simulink model "PubIfDecisionTOS_MDL"  (R2020b)
settings: configuration reference "DspaceConfig" (kept outside this file)
PostLoadFcn:
  | if any(exist('dsrtsu_mdlpostloadfcn', 'file') ~= 0), dsrtsu_mdlpostloadfcn('Execute', bdroot); end
InitFcn:
  | , if any(exist('dsmpb_private', 'file') ~= 0), dsmpb_private('dsmpb_mdlclblib', 'Init', bdroot); end,
undefined symbols (not defined in the file or in its folder): C_TOS_ACCEgoRAxletoFbumplength_m, C_TOS_ACCTargetFront_Flag, C_TOS_AEBJAPedObjDxThre_Val, C_TOS_AEBJAPedObjDyThre_Val, C_TOS_AEBJATargetSize_Val, C_TOS_AEBJAVehObjDxThre_Val, C_TOS_AEBJAVehObjDyThre_Val, C_TOS_AEBJuncPedTargetSize_Val, C_TOS_AEBLatObjDxThre_Val, C_TOS_AEBLatPedDyThre_Val, C_TOS_AEBLatTargetSize_Val, C_TOS_AEBLongTargetInEgoFront_Flag, C_TOS_axAbsGround_Parameter, C_TOS_CameraConfirmedFlag, C_TOS_CNsubjWidth, C_TOS_CurrentLaneCoreMinWidth_Val, C_TOS_CutInProb_Val_Zero, C_TOS_CutOutProb_Val_Zero, C_TOS_D2R_Val, C_TOS_DefaultValueObjectToCenterLine_dy, C_TOS_EgoCarWidth_Val, C_TOS_EgoDxRefPoint_m, C_TOS_EgoRAxletoFbumplength_m, C_TOS_HalfWidthVehicle_Con, C_TOS_HWA_CurrentLaneFlag, C_TOS_HWA_LeftLaneFlag, C_TOS_HWA_MovingDir_Vaild, C_TOS_HWA_MovState_Vaild, C_TOS_HWA_RightLaneFlag, C_TOS_LaneLineCourseErrorFront, C_TOS_LaneLineCourseErrorRear, C_TOS_MotorbikeDefaultWidth_m, C_TOS_NumberOfEffectiveTargets, C_TOS_Obj_Age_Val, C_TOS_Objdx_Constraint_Val, C_TOS_ObjectDefaultWidth_m, C_TOS_ObjInCurrentLane_Val, C_TOS_ObjInCurrentLaneValid, C_TOS_ObjInLeftLaneValid, C_TOS_ObjInRightLaneValid, C_TOS_ObjNotInCurrentLane_Val, C_TOS_ObjNotREElementType, C_TOS_ObjPredictDis_dy_ConstantVal_Zeros, C_TOS_ObjToCenterLine_ConstantVal_Zeros, C_TOS_OFMObjIDInvilad_Val, C_TOS_PIL_LatDisCons_Val_zero, C_TOS_PIL_ObjectCutInFlag_b, C_TOS_PIL_ObjectCutOutFlag_b, C_TOS_PIL_ObjLaneProb_al_Val, C_TOS_PP_ObjFusType_FC_Confirm_b, C_TOS_PP_ObjFusType_FC_FR_Confirm_b, C_TOS_PP_ObjFusType_FR_Confirm_b, C_TOS_RE_80BoolDefault_Val, C_TOS_RE_80Single181Default_Val, C_TOS_RE_80Single255Default_Val, C_TOS_RE_80Uint8Default_Val, C_TOS_RE_D2R, C_TOS_RE_D_180_Val, C_TOS_RE_InvalidObjectID_Val, C_TOS_RE_InvalidTargetChainDir_Val ... (+142)
libraries: simulink x1650, TOS_LIB x361, canfdmsglib x14
(part 16 of 69)

== system PubIfDecisionTOS_MDL/TOS_20201112/TOS_2012080320/PP1128/AAT-AdditionalAttributes/PP_CenterLine_Calculat/LaneWidth/Subsystem ==
  LaneWidth_FiltK1 : Inport
  LaneWidth : Inport  Port=2
  Add1 : Sum  OutDataTypeStr=single
  Add2 : Sum  Inputs=-+  OutDataTypeStr=single
  Constant : Constant  Value=P_TOS_LaneWidthFiltFactor_Val  OutDataTypeStr=single
      settings: AttributesFormatString=P_TOS_LaneWidthFiltFactor_Val = 0.2
  Product : Product  OutDataTypeStr=single
  LaneWidth_Filt : Outport
  wires:
  Constant/1 -> Product/2  "factor"
  Product/1 -> Add1/2
  Add1/1 -> LaneWidth_Filt/1  "LaneWidth_Filt"
  LaneWidth/1 -> Add2/2  "LaneWidth"
  Add2/1 -> Product/1
  LaneWidth_FiltK1/1 -> Add2/1, Add1/1

== system PubIfDecisionTOS_MDL/TOS_20201112/TOS_2012080320/PP1128/AAT-AdditionalAttributes/PP_CenterLine_Calculat/LaneWidth_80/LaneWidth ==
  TOS_OFMObjValid_Flag : Inport  Partition=on  PartitionDimension=1  PartitionWidth=1  PartitionOffset=0
  Object_MovingState : Inport  Port=2  Partition=on  PartitionDimension=1  PartitionWidth=1  PartitionOffset=0
  Object_Type : Inport  Port=3  Partition=on  PartitionDimension=1  PartitionWidth=1  PartitionOffset=0
  LM_LL_pC0 : Inport  Port=4
  LM_LR_pC0 : Inport  Port=5
  LM_RL_pC0 : Inport  Port=6
  LM_RR_pC0 : Inport  Port=7
  Bus Creator : BusCreator  Inputs=4
  Compare To Constant : simulink/Logic and Bit Operations/Compare To Constant  relop=~=  const=C_TOS_OFMObjIDInvilad_Val  OutDataTypeStr=boolean
      settings: AttributesFormatString=C_TOS_OFMObjIDInvilad_Val = 0
  Compare To Constant1 : simulink/Logic and Bit Operations/Compare To Constant  relop===  const=OFM_OBJ_TYPE_E.UNKNOWN_TYPE  OutDataTypeStr=boolean
      settings: AttributesFormatString=OFM_OBJ_TYPE_E.UNKNOWN_TYPE = 1
  Compare To Constant3 : simulink/Logic and Bit Operations/Compare To Constant  relop===  const=OFM_OBJ_MOVINGSTATE_E.STATIONARY  OutDataTypeStr=boolean
      settings: AttributesFormatString=OFM_OBJ_MOVINGSTATE_E.STATIONARY = 3
  Compare To Constant4 : simulink/Logic and Bit Operations/Compare To Constant  relop===  const=OFM_OBJ_MOVINGSTATE_E.UNKNOWN  OutDataTypeStr=boolean
      settings: AttributesFormatString=OFM_OBJ_MOVINGSTATE_E.UNKNOWN = 1
  Data Type Conversion1 : DataTypeConversion  OutDataTypeStr=Enum: OFM_OBJ_MOVINGSTATE_E
  Data Type Conversion2 : DataTypeConversion  OutDataTypeStr=Enum: OFM_OBJ_TYPE_E
  For Each : ForEach  DisableCoverage=on
  If : If  NumInputs=2  IfExpression=u1==1 & u2==1  ElseIfExpressions=u1==1 & u2==0
  Logical Operator2 : Logic  Operator=OR  AllPortsSameDT=off  OutDataTypeStr=boolean
  Merge : Merge  Inputs=3
  Merge3 : Merge  Inputs=3
  Merge4 : Merge  Inputs=3
  PP_LaneWidth : Subsystem
  PP_LaneWidthDefalut : Subsystem  TreatAsAtomicUnit=on
  PP_StaticObj_LaneWidth : Subsystem
  Terminator : Terminator
  TOS_PP_CurrentLaneWidth : Outport  ConcatenationDimension=1
  TOS_PP_LeftLaneWidth : Outport  Port=2  ConcatenationDimension=1
  TOS_PP_RightLaneWidth : Outport  Port=3  ConcatenationDimension=1
  wires:
  Bus Creator/1 -> PP_StaticObj_LaneWidth/1(LM_SignalVerification), PP_LaneWidth/1(LM_SignalVerification)
  LM_RR_pC0/1 -> Bus Creator/4  "LM_RR_pC0"
  LM_RL_pC0/1 -> Bus Creator/3  "LM_RL_pC0"
  LM_LR_pC0/1 -> Bus Creator/2  "LM_LR_pC0"
  LM_LL_pC0/1 -> Bus Creator/1  "LM_LL_pC0"
  Merge4/1 -> TOS_PP_RightLaneWidth/1
  Merge3/1 -> TOS_PP_CurrentLaneWidth/1
  PP_LaneWidthDefalut/3(TOS_PP_RightLaneWidth) -> Merge4/3
  PP_LaneWidth/3(TOS_PP_RightLaneWidth) -> Merge4/2
  PP_StaticObj_LaneWidth/3(TOS_PP_RightLaneWidth) -> Merge4/1
  PP_LaneWidthDefalut/2(TOS_PP_CurrentLaneWidth) -> Merge3/3
  PP_LaneWidth/2(TOS_PP_CurrentLaneWidth) -> Merge3/2
  PP_StaticObj_LaneWidth/2(TOS_PP_CurrentLaneWidth) -> Merge3/1
  Merge/1 -> TOS_PP_LeftLaneWidth/1
  PP_LaneWidthDefalut/1(TOS_PP_LeftLaneWidth) -> Merge/3
  PP_LaneWidth/1(TOS_PP_LeftLaneWidth) -> Merge/2
  PP_StaticObj_LaneWidth/1(TOS_PP_LeftLaneWidth) -> Merge/1
  If/3 -> PP_LaneWidthDefalut/Action
  If/2 -> PP_LaneWidth/Action
  Compare To Constant3/1 -> Logical Operator2/1
  Logical Operator2/1 -> If/2
  Object_MovingState/1 -> Data Type Conversion1/1
  Object_Type/1 -> Data Type Conversion2/1
  Data Type Conversion1/1 -> Compare To Constant4/1, Compare To Constant3/1
  Data Type Conversion2/1 -> Compare To Constant1/1
  Compare To Constant1/1 -> Terminator/1
  Compare To Constant4/1 -> Logical Operator2/2
  Compare To Constant/1 -> If/1
  If/1 -> PP_StaticObj_LaneWidth/Action
  TOS_OFMObjValid_Flag/1 -> Compare To Constant/1

== system PubIfDecisionTOS_MDL/TOS_20201112/TOS_2012080320/PP1128/AAT-AdditionalAttributes/PP_CenterLine_Calculat/LeftLane_CenterLine/LaneCenterLine01 ==
  LaneLine : Inport
  Add{,1..3} (4 alike) : Sum
  Bus Creator : BusCreator  Inputs=6
  Bus Selector : BusSelector  OutputSignals=TOS_LM_LL_Bus.LM_LL_Line01.pC0,TOS_LM_LR_Bus.LM_LR_Line01.pC0
  Bus Selector1 : BusSelector  OutputSignals=TOS_LM_LL_Bus.LM_LL_Line01.pC3,TOS_LM_LR_Bus.LM_LR_Line01.pC3
  Bus Selector2 : BusSelector  OutputSignals=TOS_LM_LL_Bus.LM_LL_Line01.pC2,TOS_LM_LR_Bus.LM_LR_Line01.pC2
  Bus Selector3 : BusSelector  OutputSignals=TOS_LM_LL_Bus.LM_LL_Line01.pC1,TOS_LM_LR_Bus.LM_LR_Line01.pC1
  Bus Selector4 : BusSelector  OutputSignals=TOS_LM_LL_Bus.LM_LL_Line01.dDisStart,TOS_LM_LL_Bus.LM_LL_Line01.dDisEnd
  Data{,1..3} (4 alike) : TOS_LIB/Data  SystemSampleTime=-1  VariantActivationTime=update diagram  Latency=0  AutoFrameSizeCalculation=off
  Gain{1..4} (4 alike) : Gain  Gain=0.5  ParamDataTypeStr=single  OutDataTypeStr=single
  Signal Copy1 : SignalConversion  OverrideOpt=off
  Signal Copy2 : SignalConversion  OverrideOpt=off
  LaneCenterLine01 : Outport
  wires:
  LaneLine/1 -> Bus Selector2/1, Bus Selector3/1, Bus Selector4/1, Bus Selector/1, Bus Selector1/1
  Bus Creator/1 -> LaneCenterLine01/1  "CenterLine01"
  Bus Selector1/2 -> Add1/2  "<pC3>"
  Add1/1 -> Gain1/1
  Data3/1 -> Bus Creator/4  "PC0"
  Gain2/1 -> Data1/1  "PC2"
  Gain3/1 -> Data2/1  "PC1"
  Add/1 -> Gain4/1
  Signal Copy1/1 -> Bus Creator/6, Data3/3, Data2/3, Data1/3, Data/3  "dDisEnd"
  Bus Selector/1 -> Add/1  "<pC0>"
  Bus Selector4/1 -> Signal Copy2/1  "<dDisStart>"
  Add2/1 -> Gain2/1
  Gain1/1 -> Data/1  "PC3"
  Data1/1 -> Bus Creator/2  "PC2"
  Gain4/1 -> Data3/1  "PC0"
  Bus Selector/2 -> Add/2  "<pC0>"
  Signal Copy2/1 -> Bus Creator/5, Data3/2, Data1/2, Data/2, Data2/2  "dDisStart"
  Add3/1 -> Gain3/1
  Bus Selector3/2 -> Add3/2  "<pC1>"
  Bus Selector2/1 -> Add2/1  "<pC2>"
  Bus Selector4/2 -> Signal Copy1/1  "<dDisEnd>"
  Bus Selector2/2 -> Add2/2  "<pC2>"
  Data/1 -> Bus Creator/1  "PC3"
  Bus Selector3/1 -> Add3/1  "<pC1>"
  Data2/1 -> Bus Creator/3  "PC1"
  Bus Selector1/1 -> Add1/1  "<pC3>"

== system PubIfDecisionTOS_MDL/TOS_20201112/TOS_2012080320/PP1128/AAT-AdditionalAttributes/PP_CenterLine_Calculat/LeftLane_CenterLine/LaneCenterLine02 ==
  LaneLine : Inport
  Add{,1..3} (4 alike) : Sum
  Bus Creator : BusCreator  Inputs=6
  Bus Selector : BusSelector  OutputSignals=TOS_LM_LL_Bus.LM_LL_Line02.pC0,TOS_LM_LR_Bus.LM_LR_Line02.pC0
  Bus Selector1 : BusSelector  OutputSignals=TOS_LM_LL_Bus.LM_LL_Line02.pC3,TOS_LM_LR_Bus.LM_LR_Line02.pC3
  Bus Selector2 : BusSelector  OutputSignals=TOS_LM_LL_Bus.LM_LL_Line02.pC2,TOS_LM_LR_Bus.LM_LR_Line02.pC2
  Bus Selector3 : BusSelector  OutputSignals=TOS_LM_LL_Bus.LM_LL_Line02.pC1,TOS_LM_LR_Bus.LM_LR_Line02.pC1
  Bus Selector4 : BusSelector  OutputSignals=TOS_LM_LL_Bus.LM_LL_Line02.dDisStart,TOS_LM_LL_Bus.LM_LL_Line02.dDisEnd
  Data{,1..3} (4 alike) : TOS_LIB/Data  SystemSampleTime=-1  VariantActivationTime=update diagram  Latency=0  AutoFrameSizeCalculation=off
  Gain{1..4} (4 alike) : Gain  Gain=0.5  ParamDataTypeStr=single  OutDataTypeStr=single
  Signal Copy1 : SignalConversion  OverrideOpt=off
  Signal Copy2 : SignalConversion  OverrideOpt=off
  LaneCenterLine02 : Outport
  wires:
  LaneLine/1 -> Bus Selector1/1, Bus Selector2/1, Bus Selector3/1, Bus Selector4/1, Bus Selector/1
  Bus Creator/1 -> LaneCenterLine02/1
  Bus Selector1/2 -> Add1/2  "<pC3>"
  Add1/1 -> Gain1/1
  Data3/1 -> Bus Creator/4  "PC0"
  Gain2/1 -> Data1/1  "PC2"
  Gain3/1 -> Data2/1  "PC1"
  Add/1 -> Gain4/1
  Signal Copy1/1 -> Bus Creator/6, Data3/3, Data2/3, Data1/3, Data/3  "dDisEnd"
  Bus Selector/1 -> Add/1  "<pC0>"
  Bus Selector4/1 -> Signal Copy2/1  "<dDisStart>"
  Add2/1 -> Gain2/1
  Gain1/1 -> Data/1  "PC3"
  Data1/1 -> Bus Creator/2  "PC2"
  Gain4/1 -> Data3/1  "PC0"
  Bus Selector/2 -> Add/2  "<pC0>"
  Signal Copy2/1 -> Bus Creator/5, Data3/2, Data1/2, Data/2, Data2/2  "dDisStart"
  Add3/1 -> Gain3/1
  Bus Selector3/2 -> Add3/2  "<pC1>"
  Bus Selector2/1 -> Add2/1  "<pC2>"
  Bus Selector4/2 -> Signal Copy1/1  "<dDisEnd>"
  Bus Selector2/2 -> Add2/2  "<pC2>"
  Data/1 -> Bus Creator/1  "PC3"
  Bus Selector3/1 -> Add3/1  "<pC1>"
  Data2/1 -> Bus Creator/3  "PC1"
  Bus Selector1/1 -> Add1/1  "<pC3>"

== system PubIfDecisionTOS_MDL/TOS_20201112/TOS_2012080320/PP1128/AAT-AdditionalAttributes/PP_CenterLine_Calculat/LeftLane_CenterLine/LaneCenterLine03 ==
  LaneLine : Inport
  Add{,1..3} (4 alike) : Sum
  Bus Creator1 : BusCreator  Inputs=6
  Bus Selector : BusSelector  OutputSignals=TOS_LM_LL_Bus.LM_LL_Line03.pC0,TOS_LM_LR_Bus.LM_LR_Line03.pC0
  Bus Selector1 : BusSelector  OutputSignals=TOS_LM_LL_Bus.LM_LL_Line03.pC3,TOS_LM_LR_Bus.LM_LR_Line03.pC3
  Bus Selector2 : BusSelector  OutputSignals=TOS_LM_LL_Bus.LM_LL_Line03.pC2,TOS_LM_LR_Bus.LM_LR_Line03.pC2
  Bus Selector3 : BusSelector  OutputSignals=TOS_LM_LL_Bus.LM_LL_Line03.pC1,TOS_LM_LR_Bus.LM_LR_Line03.pC1
  Bus Selector4 : BusSelector  OutputSignals=TOS_LM_LL_Bus.LM_LL_Line03.dDisStart,TOS_LM_LL_Bus.LM_LL_Line03.dDisEnd
  Data{,1..3} (4 alike) : TOS_LIB/Data  SystemSampleTime=-1  VariantActivationTime=update diagram  Latency=0  AutoFrameSizeCalculation=off
  Gain{1..4} (4 alike) : Gain  Gain=0.5  ParamDataTypeStr=single  OutDataTypeStr=single
  Signal Copy1 : SignalConversion  OverrideOpt=off
  Signal Copy2 : SignalConversion  OverrideOpt=off
  LaneCenterLine03 : Outport
  wires:
  LaneLine/1 -> Bus Selector1/1, Bus Selector2/1, Bus Selector3/1, Bus Selector4/1, Bus Selector/1
  Bus Creator1/1 -> LaneCenterLine03/1
  Bus Selector1/2 -> Add1/2  "<pC3>"
  Add1/1 -> Gain1/1
  Data3/1 -> Bus Creator1/4  "PC0"
  Gain2/1 -> Data1/1  "PC2"
  Gain3/1 -> Data2/1  "PC1"
  Add/1 -> Gain4/1
  Signal Copy1/1 -> Bus Creator1/6, Data3/3, Data2/3, Data1/3, Data/3  "dDisEnd"
  Bus Selector/1 -> Add/1  "<pC0>"
  Bus Selector4/1 -> Signal Copy2/1  "<dDisStart>"
  Add2/1 -> Gain2/1
  Gain1/1 -> Data/1  "PC3"
  Data1/1 -> Bus Creator1/2  "PC2"
  Gain4/1 -> Data3/1  "PC0"
  Bus Selector/2 -> Add/2  "<pC0>"
  Signal Copy2/1 -> Bus Creator1/5, Data3/2, Data1/2, Data/2, Data2/2  "dDisStart"
  Add3/1 -> Gain3/1
  Bus Selector3/2 -> Add3/2  "<pC1>"
  Bus Selector2/1 -> Add2/1  "<pC2>"
  Bus Selector4/2 -> Signal Copy1/1  "<dDisEnd>"
  Bus Selector2/2 -> Add2/2  "<pC2>"
  Data/1 -> Bus Creator1/1  "PC3"
  Bus Selector3/1 -> Add3/1  "<pC1>"
  Data2/1 -> Bus Creator1/3  "PC1"
  Bus Selector1/1 -> Add1/1  "<pC3>"

== system PubIfDecisionTOS_MDL/TOS_20201112/TOS_2012080320/PP1128/AAT-AdditionalAttributes/PP_CenterLine_Calculat/LeftLane_CenterLine/LaneCenterLine04 ==
  LaneLine : Inport
  Add{,1..3} (4 alike) : Sum
  Bus Creator1 : BusCreator  Inputs=6
  Bus Selector : BusSelector  OutputSignals=TOS_LM_LL_Bus.LM_LL_Line04.pC0,TOS_LM_LR_Bus.LM_LR_Line04.pC0
  Bus Selector1 : BusSelector  OutputSignals=TOS_LM_LL_Bus.LM_LL_Line04.pC3,TOS_LM_LR_Bus.LM_LR_Line04.pC3
  Bus Selector2 : BusSelector  OutputSignals=TOS_LM_LL_Bus.LM_LL_Line04.pC2,TOS_LM_LR_Bus.LM_LR_Line04.pC2
  Bus Selector3 : BusSelector  OutputSignals=TOS_LM_LL_Bus.LM_LL_Line04.pC1,TOS_LM_LR_Bus.LM_LR_Line04.pC1
  Bus Selector4 : BusSelector  OutputSignals=TOS_LM_LL_Bus.LM_LL_Line04.dDisStart,TOS_LM_LL_Bus.LM_LL_Line04.dDisEnd
  Data{,1..3} (4 alike) : TOS_LIB/Data  SystemSampleTime=-1  VariantActivationTime=update diagram  Latency=0  AutoFrameSizeCalculation=off
  Gain{1..4} (4 alike) : Gain  Gain=0.5  ParamDataTypeStr=single  OutDataTypeStr=single
  Signal Copy1 : SignalConversion  OverrideOpt=off
  Signal Copy2 : SignalConversion  OverrideOpt=off
  LaneCenterLine04 : Outport
  wires:
  LaneLine/1 -> Bus Selector1/1, Bus Selector2/1, Bus Selector3/1, Bus Selector4/1, Bus Selector/1
  Bus Creator1/1 -> LaneCenterLine04/1
  Bus Selector1/2 -> Add1/2  "<pC3>"
  Add1/1 -> Gain1/1
  Data3/1 -> Bus Creator1/4  "PC0"
  Gain2/1 -> Data1/1  "PC2"
  Gain3/1 -> Data2/1  "PC1"
  Add/1 -> Gain4/1
  Signal Copy1/1 -> Bus Creator1/6, Data3/3, Data2/3, Data1/3, Data/3  "dDisEnd"
  Bus Selector/1 -> Add/1  "<pC0>"
  Bus Selector4/1 -> Signal Copy2/1  "<dDisStart>"
  Add2/1 -> Gain2/1
  Gain1/1 -> Data/1  "PC3"
  Data1/1 -> Bus Creator1/2  "PC2"
  Gain4/1 -> Data3/1  "PC0"
  Bus Selector/2 -> Add/2  "<pC0>"
  Signal Copy2/1 -> Bus Creator1/5, Data3/2, Data1/2, Data/2, Data2/2  "dDisStart"
  Add3/1 -> Gain3/1
  Bus Selector3/2 -> Add3/2  "<pC1>"
  Bus Selector2/1 -> Add2/1  "<pC2>"
  Bus Selector4/2 -> Signal Copy1/1  "<dDisEnd>"
  Bus Selector2/2 -> Add2/2  "<pC2>"
  Data/1 -> Bus Creator1/1  "PC3"
  Bus Selector3/1 -> Add3/1  "<pC1>"
  Data2/1 -> Bus Creator1/3  "PC1"
  Bus Selector1/1 -> Add1/1  "<pC3>"

== system PubIfDecisionTOS_MDL/TOS_20201112/TOS_2012080320/PP1128/AAT-AdditionalAttributes/PP_CenterLine_Calculat/LeftLane_CenterLine/LaneCenterLine05 ==
  LaneLine : Inport
  Add{,1..3} (4 alike) : Sum
  Bus Creator1 : BusCreator  Inputs=6
  Bus Selector : BusSelector  OutputSignals=TOS_LM_LL_Bus.LM_LL_Line05.pC0,TOS_LM_LR_Bus.LM_LR_Line05.pC0
  Bus Selector1 : BusSelector  OutputSignals=TOS_LM_LL_Bus.LM_LL_Line05.pC3,TOS_LM_LR_Bus.LM_LR_Line05.pC3
  Bus Selector2 : BusSelector  OutputSignals=TOS_LM_LL_Bus.LM_LL_Line05.pC2,TOS_LM_LR_Bus.LM_LR_Line05.pC2
  Bus Selector3 : BusSelector  OutputSignals=TOS_LM_LL_Bus.LM_LL_Line05.pC1,TOS_LM_LR_Bus.LM_LR_Line05.pC1
  Bus Selector4 : BusSelector  OutputSignals=TOS_LM_LL_Bus.LM_LL_Line05.dDisStart,TOS_LM_LL_Bus.LM_LL_Line05.dDisEnd
  Data{,1..3} (4 alike) : TOS_LIB/Data  SystemSampleTime=-1  VariantActivationTime=update diagram  Latency=0  AutoFrameSizeCalculation=off
  Gain{1..4} (4 alike) : Gain  Gain=0.5  ParamDataTypeStr=single  OutDataTypeStr=single
  Signal Copy1 : SignalConversion  OverrideOpt=off
  Signal Copy2 : SignalConversion  OverrideOpt=off
  LaneCenterLine05 : Outport
  wires:
  Bus Creator1/1 -> LaneCenterLine05/1
  LaneLine/1 -> Bus Selector1/1, Bus Selector2/1, Bus Selector4/1, Bus Selector/1, Bus Selector3/1
  Bus Selector1/2 -> Add1/2  "<pC3>"
  Add1/1 -> Gain1/1
  Data3/1 -> Bus Creator1/4  "PC0"
  Gain2/1 -> Data1/1  "PC2"
  Gain3/1 -> Data2/1  "PC1"
  Add/1 -> Gain4/1
  Signal Copy1/1 -> Data3/3, Data2/3, Data1/3, Data/3, Bus Creator1/6  "dDisEnd"
  Bus Selector/1 -> Add/1  "<pC0>"
  Bus Selector4/1 -> Signal Copy2/1  "<dDisStart>"
  Add2/1 -> Gain2/1
  Gain1/1 -> Data/1  "PC3"
  Data1/1 -> Bus Creator1/2  "PC2"
  Gain4/1 -> Data3/1  "PC0"
  Bus Selector/2 -> Add/2  "<pC0>"
  Signal Copy2/1 -> Data3/2, Data1/2, Data/2, Data2/2, Bus Creator1/5  "dDisStart"
  Add3/1 -> Gain3/1
  Bus Selector3/2 -> Add3/2  "<pC1>"
  Bus Selector2/1 -> Add2/1  "<pC2>"
  Bus Selector4/2 -> Signal Copy1/1  "<dDisEnd>"
  Bus Selector2/2 -> Add2/2  "<pC2>"
  Data/1 -> Bus Creator1/1  "PC3"
  Bus Selector3/1 -> Add3/1  "<pC1>"
  Data2/1 -> Bus Creator1/3  "PC1"
  Bus Selector1/1 -> Add1/1  "<pC3>"

== system PubIfDecisionTOS_MDL/TOS_20201112/TOS_2012080320/PP1128/AAT-AdditionalAttributes/PP_CenterLine_Calculat/LeftLane_CenterLine/LaneCenterLine06 ==
  LaneLine : Inport
  Add{,1..3} (4 alike) : Sum
  Bus Creator1 : BusCreator  Inputs=6
  Bus Selector : BusSelector  OutputSignals=TOS_LM_LL_Bus.LM_LL_Line06.pC0,TOS_LM_LR_Bus.LM_LR_Line06.pC0
  Bus Selector1 : BusSelector  OutputSignals=TOS_LM_LL_Bus.LM_LL_Line06.pC3,TOS_LM_LR_Bus.LM_LR_Line06.pC3
  Bus Selector2 : BusSelector  OutputSignals=TOS_LM_LL_Bus.LM_LL_Line06.pC2,TOS_LM_LR_Bus.LM_LR_Line06.pC2
  Bus Selector3 : BusSelector  OutputSignals=TOS_LM_LL_Bus.LM_LL_Line06.pC1,TOS_LM_LR_Bus.LM_LR_Line06.pC1
  Bus Selector4 : BusSelector  OutputSignals=TOS_LM_LL_Bus.LM_LL_Line06.dDisStart,TOS_LM_LL_Bus.LM_LL_Line06.dDisEnd
  Data{,1..3} (4 alike) : TOS_LIB/Data  SystemSampleTime=-1  VariantActivationTime=update diagram  Latency=0  AutoFrameSizeCalculation=off
  Gain{1..4} (4 alike) : Gain  Gain=0.5  ParamDataTypeStr=single  OutDataTypeStr=single
  Signal Copy1 : SignalConversion  OverrideOpt=off
  Signal Copy2 : SignalConversion  OverrideOpt=off
  LaneCenterLine06 : Outport
  wires:
  Bus Creator1/1 -> LaneCenterLine06/1
  LaneLine/1 -> Bus Selector1/1, Bus Selector2/1, Bus Selector3/1, Bus Selector4/1, Bus Selector/1
  Bus Selector1/2 -> Add1/2  "<pC3>"
  Add1/1 -> Gain1/1
  Data3/1 -> Bus Creator1/4  "PC0"
  Gain2/1 -> Data1/1  "PC2"
  Gain3/1 -> Data2/1  "PC1"
  Add/1 -> Gain4/1
  Signal Copy1/1 -> Bus Creator1/6, Data3/3, Data2/3, Data1/3, Data/3  "dDisEnd"
  Bus Selector/1 -> Add/1  "<pC0>"
  Bus Selector4/1 -> Signal Copy2/1  "<dDisStart>"
  Add2/1 -> Gain2/1
  Gain1/1 -> Data/1  "PC3"
  Data1/1 -> Bus Creator1/2  "PC2"
  Gain4/1 -> Data3/1  "PC0"
  Bus Selector/2 -> Add/2  "<pC0>"
  Signal Copy2/1 -> Bus Creator1/5, Data3/2, Data2/2, Data1/2, Data/2  "dDisStart"
  Add3/1 -> Gain3/1
  Bus Selector3/2 -> Add3/2  "<pC1>"
  Bus Selector2/1 -> Add2/1  "<pC2>"
  Bus Selector4/2 -> Signal Copy1/1  "<dDisEnd>"
  Bus Selector2/2 -> Add2/2  "<pC2>"
  Data/1 -> Bus Creator1/1  "PC3"
  Bus Selector3/1 -> Add3/1  "<pC1>"
  Data2/1 -> Bus Creator1/3  "PC1"
  Bus Selector1/1 -> Add1/1  "<pC3>"

== system PubIfDecisionTOS_MDL/TOS_20201112/TOS_2012080320/PP1128/AAT-AdditionalAttributes/PP_CenterLine_Calculat/RightLane_CenterLine/LaneCenterLine01 ==
  LaneLine : Inport
  Add{,1..3} (4 alike) : Sum
  Bus Creator : BusCreator  Inputs=6
  Bus Selector : BusSelector  OutputSignals=TOS_LM_RL_Bus.LM_RL_Line01.pC0,TOS_LM_RR_Bus.LM_RR_Line01.pC0
  Bus Selector1 : BusSelector  OutputSignals=TOS_LM_RL_Bus.LM_RL_Line01.pC3,TOS_LM_RR_Bus.LM_RR_Line01.pC3
  Bus Selector2 : BusSelector  OutputSignals=TOS_LM_RL_Bus.LM_RL_Line01.pC2,TOS_LM_RR_Bus.LM_RR_Line01.pC2
  Bus Selector3 : BusSelector  OutputSignals=TOS_LM_RL_Bus.LM_RL_Line01.pC1,TOS_LM_RR_Bus.LM_RR_Line01.pC1
  Bus Selector4 : BusSelector  OutputSignals=TOS_LM_RL_Bus.LM_RL_Line01.dDisStart,TOS_LM_RL_Bus.LM_RL_Line01.dDisEnd
  Data{,1..3} (4 alike) : TOS_LIB/Data  SystemSampleTime=-1  VariantActivationTime=update diagram  Latency=0  AutoFrameSizeCalculation=off
  Gain{1..4} (4 alike) : Gain  Gain=0.5  ParamDataTypeStr=single  OutDataTypeStr=single
  Signal Copy1 : SignalConversion  OverrideOpt=off
  Signal Copy2 : SignalConversion  OverrideOpt=off
  LaneCenterLine01 : Outport
  wires:
  LaneLine/1 -> Bus Selector2/1, Bus Selector3/1, Bus Selector4/1, Bus Selector/1, Bus Selector1/1
  Bus Creator/1 -> LaneCenterLine01/1  "CenterLine01"
  Bus Selector1/2 -> Add1/2  "<pC3>"
  Add1/1 -> Gain1/1
  Data3/1 -> Bus Creator/4  "PC0"
  Gain2/1 -> Data1/1  "PC2"
  Gain3/1 -> Data2/1  "PC1"
  Add/1 -> Gain4/1
  Signal Copy1/1 -> Bus Creator/6, Data3/3, Data2/3, Data/3, Data1/3  "dDisEnd"
  Bus Selector/1 -> Add/1  "<pC0>"
  Bus Selector4/1 -> Signal Copy2/1  "<dDisStart>"
  Add2/1 -> Gain2/1
  Gain1/1 -> Data/1  "PC3"
  Data1/1 -> Bus Creator/2  "PC2"
  Gain4/1 -> Data3/1  "PC0"
  Bus Selector/2 -> Add/2  "<pC0>"
  Signal Copy2/1 -> Bus Creator/5, Data3/2, Data2/2, Data/2, Data1/2  "dDisStart"
  Add3/1 -> Gain3/1
  Bus Selector3/2 -> Add3/2  "<pC1>"
  Bus Selector2/1 -> Add2/1  "<pC2>"
  Bus Selector4/2 -> Signal Copy1/1  "<dDisEnd>"
  Bus Selector2/2 -> Add2/2  "<pC2>"
  Data/1 -> Bus Creator/1  "PC3"
  Bus Selector3/1 -> Add3/1  "<pC1>"
  Data2/1 -> Bus Creator/3  "PC1"
  Bus Selector1/1 -> Add1/1  "<pC3>"

== system PubIfDecisionTOS_MDL/TOS_20201112/TOS_2012080320/PP1128/AAT-AdditionalAttributes/PP_CenterLine_Calculat/RightLane_CenterLine/LaneCenterLine02 ==
  LaneLine : Inport
  Add{,1..3} (4 alike) : Sum
  Bus Creator : BusCreator  Inputs=6
  Bus Selector : BusSelector  OutputSignals=TOS_LM_RL_Bus.LM_RL_Line02.pC0,TOS_LM_RR_Bus.LM_RR_Line02.pC0
  Bus Selector1 : BusSelector  OutputSignals=TOS_LM_RL_Bus.LM_RL_Line02.pC3,TOS_LM_RR_Bus.LM_RR_Line02.pC3
  Bus Selector2 : BusSelector  OutputSignals=TOS_LM_RL_Bus.LM_RL_Line02.pC2,TOS_LM_RR_Bus.LM_RR_Line02.pC2
  Bus Selector3 : BusSelector  OutputSignals=TOS_LM_RL_Bus.LM_RL_Line02.pC1,TOS_LM_RR_Bus.LM_RR_Line02.pC1
  Bus Selector4 : BusSelector  OutputSignals=TOS_LM_RL_Bus.LM_RL_Line02.dDisStart,TOS_LM_RL_Bus.LM_RL_Line02.dDisEnd
  Data{,1..3} (4 alike) : TOS_LIB/Data  SystemSampleTime=-1  VariantActivationTime=update diagram  Latency=0  AutoFrameSizeCalculation=off
  Gain{1..4} (4 alike) : Gain  Gain=0.5  ParamDataTypeStr=single  OutDataTypeStr=single
  Signal Copy1 : SignalConversion  OverrideOpt=off
  Signal Copy2 : SignalConversion  OverrideOpt=off
  LaneCenterLine02 : Outport
  wires:
  LaneLine/1 -> Bus Selector1/1, Bus Selector2/1, Bus Selector3/1, Bus Selector4/1, Bus Selector/1
  Bus Creator/1 -> LaneCenterLine02/1
  Bus Selector1/2 -> Add1/2  "<pC3>"
  Add1/1 -> Gain1/1
  Data3/1 -> Bus Creator/4  "PC0"
  Gain2/1 -> Data1/1  "PC2"
  Gain3/1 -> Data2/1  "PC1"
  Add/1 -> Gain4/1
  Signal Copy1/1 -> Bus Creator/6, Data3/3, Data2/3, Data1/3, Data/3  "dDisEnd"
  Bus Selector/1 -> Add/1  "<pC0>"
  Bus Selector4/1 -> Signal Copy2/1  "<dDisStart>"
  Add2/1 -> Gain2/1
  Gain1/1 -> Data/1  "PC3"
  Data1/1 -> Bus Creator/2  "PC2"
  Gain4/1 -> Data3/1  "PC0"
  Bus Selector/2 -> Add/2  "<pC0>"
  Signal Copy2/1 -> Bus Creator/5, Data3/2, Data2/2, Data1/2, Data/2  "dDisStart"
  Add3/1 -> Gain3/1
  Bus Selector3/2 -> Add3/2  "<pC1>"
  Bus Selector2/1 -> Add2/1  "<pC2>"
  Bus Selector4/2 -> Signal Copy1/1  "<dDisEnd>"
  Bus Selector2/2 -> Add2/2  "<pC2>"
  Data/1 -> Bus Creator/1  "PC3"
  Bus Selector3/1 -> Add3/1  "<pC1>"
  Data2/1 -> Bus Creator/3  "PC1"
  Bus Selector1/1 -> Add1/1  "<pC3>"

== system PubIfDecisionTOS_MDL/TOS_20201112/TOS_2012080320/PP1128/AAT-AdditionalAttributes/PP_CenterLine_Calculat/RightLane_CenterLine/LaneCenterLine03 ==
  LaneLine : Inport
  Add{,1..3} (4 alike) : Sum
  Bus Creator1 : BusCreator  Inputs=6
  Bus Selector : BusSelector  OutputSignals=TOS_LM_RL_Bus.LM_RL_Line03.pC0,TOS_LM_RR_Bus.LM_RR_Line03.pC0
  Bus Selector1 : BusSelector  OutputSignals=TOS_LM_RL_Bus.LM_RL_Line03.pC3,TOS_LM_RR_Bus.LM_RR_Line03.pC3
  Bus Selector2 : BusSelector  OutputSignals=TOS_LM_RL_Bus.LM_RL_Line03.pC2,TOS_LM_RR_Bus.LM_RR_Line03.pC2
  Bus Selector3 : BusSelector  OutputSignals=TOS_LM_RL_Bus.LM_RL_Line03.pC1,TOS_LM_RR_Bus.LM_RR_Line03.pC1
  Bus Selector4 : BusSelector  OutputSignals=TOS_LM_RL_Bus.LM_RL_Line03.dDisStart,TOS_LM_RL_Bus.LM_RL_Line03.dDisEnd
  Data{,1..3} (4 alike) : TOS_LIB/Data  SystemSampleTime=-1  VariantActivationTime=update diagram  Latency=0  AutoFrameSizeCalculation=off
  Gain{1..4} (4 alike) : Gain  Gain=0.5  ParamDataTypeStr=single  OutDataTypeStr=single
  Signal Copy1 : SignalConversion  OverrideOpt=off
  Signal Copy2 : SignalConversion  OverrideOpt=off
  LaneCenterLine03 : Outport
  wires:
  LaneLine/1 -> Bus Selector1/1, Bus Selector2/1, Bus Selector3/1, Bus Selector4/1, Bus Selector/1
  Bus Creator1/1 -> LaneCenterLine03/1
  Bus Selector1/2 -> Add1/2  "<pC3>"
  Add1/1 -> Gain1/1
  Data3/1 -> Bus Creator1/4  "PC0"
  Gain2/1 -> Data1/1  "PC2"
  Gain3/1 -> Data2/1  "PC1"
  Add/1 -> Gain4/1
  Signal Copy1/1 -> Bus Creator1/6, Data3/3, Data2/3, Data1/3, Data/3  "dDisEnd"
  Bus Selector/1 -> Add/1  "<pC0>"
  Bus Selector4/1 -> Signal Copy2/1  "<dDisStart>"
  Add2/1 -> Gain2/1
  Gain1/1 -> Data/1  "PC3"
  Data1/1 -> Bus Creator1/2  "PC2"
  Gain4/1 -> Data3/1  "PC0"
  Bus Selector/2 -> Add/2  "<pC0>"
  Signal Copy2/1 -> Bus Creator1/5, Data3/2, Data2/2, Data1/2, Data/2  "dDisStart"
  Add3/1 -> Gain3/1
  Bus Selector3/2 -> Add3/2  "<pC1>"
  Bus Selector2/1 -> Add2/1  "<pC2>"
  Bus Selector4/2 -> Signal Copy1/1  "<dDisEnd>"
  Bus Selector2/2 -> Add2/2  "<pC2>"
  Data/1 -> Bus Creator1/1  "PC3"
  Bus Selector3/1 -> Add3/1  "<pC1>"
  Data2/1 -> Bus Creator1/3  "PC1"
  Bus Selector1/1 -> Add1/1  "<pC3>"

== system PubIfDecisionTOS_MDL/TOS_20201112/TOS_2012080320/PP1128/AAT-AdditionalAttributes/PP_CenterLine_Calculat/RightLane_CenterLine/LaneCenterLine04 ==
  LaneLine : Inport
  Add{,1..3} (4 alike) : Sum
  Bus Creator1 : BusCreator  Inputs=6
  Bus Selector : BusSelector  OutputSignals=TOS_LM_RL_Bus.LM_RL_Line04.pC0,TOS_LM_RR_Bus.LM_RR_Line04.pC0
  Bus Selector1 : BusSelector  OutputSignals=TOS_LM_RL_Bus.LM_RL_Line04.pC3,TOS_LM_RR_Bus.LM_RR_Line04.pC3
  Bus Selector2 : BusSelector  OutputSignals=TOS_LM_RL_Bus.LM_RL_Line04.pC2,TOS_LM_RR_Bus.LM_RR_Line04.pC2
  Bus Selector3 : BusSelector  OutputSignals=TOS_LM_RL_Bus.LM_RL_Line04.pC1,TOS_LM_RR_Bus.LM_RR_Line04.pC1
  Bus Selector4 : BusSelector  OutputSignals=TOS_LM_RL_Bus.LM_RL_Line04.dDisStart,TOS_LM_RL_Bus.LM_RL_Line04.dDisEnd
  Data{,1..3} (4 alike) : TOS_LIB/Data  SystemSampleTime=-1  VariantActivationTime=update diagram  Latency=0  AutoFrameSizeCalculation=off
  Gain{1..4} (4 alike) : Gain  Gain=0.5  ParamDataTypeStr=single  OutDataTypeStr=single
  Signal Copy1 : SignalConversion  OverrideOpt=off
  Signal Copy2 : SignalConversion  OverrideOpt=off
  LaneCenterLine04 : Outport
  wires:
  LaneLine/1 -> Bus Selector1/1, Bus Selector2/1, Bus Selector3/1, Bus Selector4/1, Bus Selector/1
  Bus Creator1/1 -> LaneCenterLine04/1
  Bus Selector1/2 -> Add1/2  "<pC3>"
  Add1/1 -> Gain1/1
  Data3/1 -> Bus Creator1/4  "PC0"
  Gain2/1 -> Data1/1  "PC2"
  Gain3/1 -> Data2/1  "PC1"
  Add/1 -> Gain4/1
  Signal Copy1/1 -> Bus Creator1/6, Data3/3, Data2/3, Data/3, Data1/3  "dDisEnd"
  Bus Selector/1 -> Add/1  "<pC0>"
  Bus Selector4/1 -> Signal Copy2/1  "<dDisStart>"
  Add2/1 -> Gain2/1
  Gain1/1 -> Data/1  "PC3"
  Data1/1 -> Bus Creator1/2  "PC2"
  Gain4/1 -> Data3/1  "PC0"
  Bus Selector/2 -> Add/2  "<pC0>"
  Signal Copy2/1 -> Bus Creator1/5, Data3/2, Data2/2, Data/2, Data1/2  "dDisStart"
  Add3/1 -> Gain3/1
  Bus Selector3/2 -> Add3/2  "<pC1>"
  Bus Selector2/1 -> Add2/1  "<pC2>"
  Bus Selector4/2 -> Signal Copy1/1  "<dDisEnd>"
  Bus Selector2/2 -> Add2/2  "<pC2>"
  Data/1 -> Bus Creator1/1  "PC3"
  Bus Selector3/1 -> Add3/1  "<pC1>"
  Data2/1 -> Bus Creator1/3  "PC1"
  Bus Selector1/1 -> Add1/1  "<pC3>"

== system PubIfDecisionTOS_MDL/TOS_20201112/TOS_2012080320/PP1128/AAT-AdditionalAttributes/PP_CenterLine_Calculat/RightLane_CenterLine/LaneCenterLine05 ==
  LaneLine : Inport
  Add{,1..3} (4 alike) : Sum
  Bus Creator1 : BusCreator  Inputs=6
  Bus Selector : BusSelector  OutputSignals=TOS_LM_RL_Bus.LM_RL_Line05.pC0,TOS_LM_RR_Bus.LM_RR_Line05.pC0
  Bus Selector1 : BusSelector  OutputSignals=TOS_LM_RL_Bus.LM_RL_Line05.pC3,TOS_LM_RR_Bus.LM_RR_Line05.pC3
  Bus Selector2 : BusSelector  OutputSignals=TOS_LM_RL_Bus.LM_RL_Line05.pC2,TOS_LM_RR_Bus.LM_RR_Line05.pC2
  Bus Selector3 : BusSelector  OutputSignals=TOS_LM_RL_Bus.LM_RL_Line05.pC1,TOS_LM_RR_Bus.LM_RR_Line05.pC1
  Bus Selector4 : BusSelector  OutputSignals=TOS_LM_RL_Bus.LM_RL_Line05.dDisStart,TOS_LM_RL_Bus.LM_RL_Line05.dDisEnd
  Data{,1..3} (4 alike) : TOS_LIB/Data  SystemSampleTime=-1  VariantActivationTime=update diagram  Latency=0  AutoFrameSizeCalculation=off
  Gain{1..4} (4 alike) : Gain  Gain=0.5  ParamDataTypeStr=single  OutDataTypeStr=single
  Signal Copy1 : SignalConversion  OverrideOpt=off
  Signal Copy2 : SignalConversion  OverrideOpt=off
  LaneCenterLine05 : Outport
  wires:
  Bus Creator1/1 -> LaneCenterLine05/1
  LaneLine/1 -> Bus Selector1/1, Bus Selector2/1, Bus Selector3/1, Bus Selector4/1, Bus Selector/1
  Bus Selector1/2 -> Add1/2  "<pC3>"
  Add1/1 -> Gain1/1
  Data3/1 -> Bus Creator1/4  "PC0"
  Gain2/1 -> Data1/1  "PC2"
  Gain3/1 -> Data2/1  "PC1"
  Add/1 -> Gain4/1
  Signal Copy1/1 -> Bus Creator1/6, Data3/3, Data2/3, Data1/3, Data/3  "dDisEnd"
  Bus Selector/1 -> Add/1  "<pC0>"
  Bus Selector4/1 -> Signal Copy2/1  "<dDisStart>"
  Add2/1 -> Gain2/1
  Gain1/1 -> Data/1  "PC3"
  Data1/1 -> Bus Creator1/2  "PC2"
  Gain4/1 -> Data3/1  "PC0"
  Bus Selector/2 -> Add/2  "<pC0>"
  Signal Copy2/1 -> Bus Creator1/5, Data3/2, Data2/2, Data1/2, Data/2  "dDisStart"
  Add3/1 -> Gain3/1
  Bus Selector3/2 -> Add3/2  "<pC1>"
  Bus Selector2/1 -> Add2/1  "<pC2>"
  Bus Selector4/2 -> Signal Copy1/1  "<dDisEnd>"
  Bus Selector2/2 -> Add2/2  "<pC2>"
  Data/1 -> Bus Creator1/1  "PC3"
  Bus Selector3/1 -> Add3/1  "<pC1>"
  Data2/1 -> Bus Creator1/3  "PC1"
  Bus Selector1/1 -> Add1/1  "<pC3>"

== system PubIfDecisionTOS_MDL/TOS_20201112/TOS_2012080320/PP1128/AAT-AdditionalAttributes/PP_CenterLine_Calculat/RightLane_CenterLine/LaneCenterLine06 ==
  LaneLine : Inport
  Add{,1..3} (4 alike) : Sum
  Bus Creator1 : BusCreator  Inputs=6
  Bus Selector : BusSelector  OutputSignals=TOS_LM_RL_Bus.LM_RL_Line06.pC0,TOS_LM_RR_Bus.LM_RR_Line06.pC0
  Bus Selector1 : BusSelector  OutputSignals=TOS_LM_RL_Bus.LM_RL_Line06.pC3,TOS_LM_RR_Bus.LM_RR_Line06.pC3
  Bus Selector2 : BusSelector  OutputSignals=TOS_LM_RL_Bus.LM_RL_Line06.pC2,TOS_LM_RR_Bus.LM_RR_Line06.pC2
  Bus Selector3 : BusSelector  OutputSignals=TOS_LM_RL_Bus.LM_RL_Line06.pC1,TOS_LM_RR_Bus.LM_RR_Line06.pC1
  Bus Selector4 : BusSelector  OutputSignals=TOS_LM_RL_Bus.LM_RL_Line06.dDisStart,TOS_LM_RL_Bus.LM_RL_Line06.dDisEnd
  Data{,1..3} (4 alike) : TOS_LIB/Data  SystemSampleTime=-1  VariantActivationTime=update diagram  Latency=0  AutoFrameSizeCalculation=off
  Gain{1..4} (4 alike) : Gain  Gain=0.5  ParamDataTypeStr=single  OutDataTypeStr=single
  Signal Copy1 : SignalConversion  OverrideOpt=off
  Signal Copy2 : SignalConversion  OverrideOpt=off
  LaneCenterLine06 : Outport
  wires:
  Bus Creator1/1 -> LaneCenterLine06/1
  LaneLine/1 -> Bus Selector1/1, Bus Selector2/1, Bus Selector3/1, Bus Selector4/1, Bus Selector/1
  Bus Selector1/2 -> Add1/2  "<pC3>"
  Add1/1 -> Gain1/1
  Data3/1 -> Bus Creator1/4  "PC0"
  Gain2/1 -> Data1/1  "PC2"
  Gain3/1 -> Data2/1  "PC1"
  Add/1 -> Gain4/1
  Signal Copy1/1 -> Bus Creator1/6, Data3/3, Data2/3, Data1/3, Data/3  "dDisEnd"
  Bus Selector/1 -> Add/1  "<pC0>"
  Bus Selector4/1 -> Signal Copy2/1  "<dDisStart>"
  Add2/1 -> Gain2/1
  Gain1/1 -> Data/1  "PC3"
  Data1/1 -> Bus Creator1/2  "PC2"
  Gain4/1 -> Data3/1  "PC0"
  Bus Selector/2 -> Add/2  "<pC0>"
  Signal Copy2/1 -> Bus Creator1/5, Data3/2, Data2/2, Data1/2, Data/2  "dDisStart"
  Add3/1 -> Gain3/1
  Bus Selector3/2 -> Add3/2  "<pC1>"
  Bus Selector2/1 -> Add2/1  "<pC2>"
  Bus Selector4/2 -> Signal Copy1/1  "<dDisEnd>"
  Bus Selector2/2 -> Add2/2  "<pC2>"
  Data/1 -> Bus Creator1/1  "PC3"
  Bus Selector3/1 -> Add3/1  "<pC1>"
  Data2/1 -> Bus Creator1/3  "PC1"
  Bus Selector1/1 -> Add1/1  "<pC3>"

== system PubIfDecisionTOS_MDL/TOS_20201112/TOS_2012080320/PP1128/AAT-AdditionalAttributes/PP_ObjFirstDxDyDetermineSignalProcessing/PP_ObjFirstDxDyDetermine/PP_ObjFirstDxDyDetermine ==
  Object_ID : Inport
  Object_Dx : Inport  Port=2
  Object_Dy : Inport  Port=3
  Object_ID_Last : Inport  Port=4
  Object_Dx_Last : Inport  Port=5
  Object_Dy_Last : Inport  Port=6
  Action Port : ActionPort  ActionPortLabel=else
  Constant : Constant  Value=C_TOS_NumberOfEffectiveTargets
      settings: AttributesFormatString=C_TOS_NumberOfEffectiveTargets = 80
  MATLAB Function : MATLAB Function  TreatAsAtomicUnit=on
  Object_ID_temp : Outport
  PP_ObjFirstDetect_Dx : Outport  Port=2
  PP_ObjFirstDetect_Dy : Outport  Port=3
  wires:
  Object_Dx_Last/1 -> MATLAB Function/5(Object_Dx_Last)
  Object_Dy_Last/1 -> MATLAB Function/6(Object_Dy_Last)
  Constant/1 -> MATLAB Function/7(C_NumberOfEffectiveTargets)
  MATLAB Function/1(Obj_DxFD) -> PP_ObjFirstDetect_Dx/1
  Object_Dx/1 -> MATLAB Function/2(Object_Dx)
  Object_ID_Last/1 -> MATLAB Function/4(Object_ID_Last)
  Object_Dy/1 -> MATLAB Function/3(Object_Dy)
  MATLAB Function/2(Obj_DyFD) -> PP_ObjFirstDetect_Dy/1
  Object_ID/1 -> Object_ID_temp/1, MATLAB Function/1(Object_ID)

== system PubIfDecisionTOS_MDL/TOS_20201112/TOS_2012080320/PP1128/AAT-AdditionalAttributes/PP_ObjFirstDxDyDetermineSignalProcessing/PP_ObjFirstDxDyDetermine/PP_ObjFirstDxDyDetermineDefault ==
  Action Port : ActionPort  ActionPortLabel=if(u1 ~= 0)
  Constant : Constant  Value=0  OutDataTypeStr=uint8
  Constant1 : Constant  Value=255  OutDataTypeStr=single
  Constant2 : Constant  Value=255  OutDataTypeStr=single
  Object_ID_temp : Outport
  PP_ObjFirstDetect_Dx : Outport  Port=2
  PP_ObjFirstDetect_Dy : Outport  Port=3
  wires:
  Constant2/1 -> PP_ObjFirstDetect_Dy/1
  Constant1/1 -> PP_ObjFirstDetect_Dx/1
  Constant/1 -> Object_ID_temp/1

== system PubIfDecisionTOS_MDL/TOS_20201112/TOS_2012080320/PP1128/AAT-AdditionalAttributes/PP_ObjectToCenterLine_dy/EgoLaneCenterLine/EgoLaneCenterLine01 ==
  EgoLaneLine : Inport
  Add{,1..3} (4 alike) : Sum
  Bus Creator : BusCreator  Inputs=6
  Bus Selector : BusSelector  OutputSignals=TOS_LM_LR_Bus.LM_LR_Line01.pC0,TOS_LM_RL_Bus.LM_RL_Line01.pC0
  Bus Selector1 : BusSelector  OutputSignals=TOS_LM_LR_Bus.LM_LR_Line01.pC3,TOS_LM_RL_Bus.LM_RL_Line01.pC3
  Bus Selector3 : BusSelector  OutputSignals=TOS_LM_LR_Bus.LM_LR_Line01.pC1,TOS_LM_RL_Bus.LM_RL_Line01.pC1
  Bus Selector4 : BusSelector  OutputSignals=TOS_LM_LR_Bus.LM_LR_Line01.dDisStart,TOS_LM_LR_Bus.LM_LR_Line01.dDisEnd
  Bus Selector5 : BusSelector  OutputSignals=TOS_LM_LR_Bus.LM_LR_Line01.pC2,TOS_LM_RL_Bus.LM_RL_Line01.pC2
  Gain{1..4} (4 alike) : Gain  Gain=0.5  ParamDataTypeStr=single  OutDataTypeStr=single
  EgoLaneCenterLine01 : Outport
  wires:
  EgoLaneLine/1 -> Bus Selector5/1, Bus Selector3/1, Bus Selector4/1, Bus Selector/1, Bus Selector1/1
  Bus Selector/1 -> Add/1  "<pC0>"
  Bus Selector/2 -> Add/2  "<pC0>"
  Add/1 -> Gain4/1
  Gain4/1 -> Bus Creator/4  "PC0"
  Add1/1 -> Gain1/1
  Bus Selector1/2 -> Add1/2  "<pC3>"
  Bus Selector1/1 -> Add1/1  "<pC3>"
  Bus Selector5/1 -> Add2/1  "<pC2>"
  Bus Selector5/2 -> Add2/2  "<pC2>"
  Add2/1 -> Gain2/1
  Add3/1 -> Gain3/1
  Bus Selector3/2 -> Add3/2  "<pC1>"
  Bus Selector3/1 -> Add3/1  "<pC1>"
  Gain1/1 -> Bus Creator/1  "PC3"
  Bus Creator/1 -> EgoLaneCenterLine01/1  "CenterLine01"
  Gain3/1 -> Bus Creator/3  "PC1"
  Gain2/1 -> Bus Creator/2  "PC2"
  Bus Selector4/1 -> Bus Creator/5  "<dDisStart>"
  Bus Selector4/2 -> Bus Creator/6  "<dDisEnd>"

== system PubIfDecisionTOS_MDL/TOS_20201112/TOS_2012080320/PP1128/AAT-AdditionalAttributes/PP_ObjectToCenterLine_dy/EgoLaneCenterLine/EgoLaneCenterLine02 ==
  EgoLaneLine : Inport
  Add{,1..3} (4 alike) : Sum
  Bus Creator : BusCreator  Inputs=6
  Bus Selector : BusSelector  OutputSignals=TOS_LM_LR_Bus.LM_LR_Line02.pC0,TOS_LM_RL_Bus.LM_RL_Line02.pC0
  Bus Selector1 : BusSelector  OutputSignals=TOS_LM_LR_Bus.LM_LR_Line02.pC3,TOS_LM_RL_Bus.LM_RL_Line02.pC3
  Bus Selector2 : BusSelector  OutputSignals=TOS_LM_LR_Bus.LM_LR_Line02.pC2,TOS_LM_RL_Bus.LM_RL_Line02.pC2
  Bus Selector3 : BusSelector  OutputSignals=TOS_LM_LR_Bus.LM_LR_Line02.pC1,TOS_LM_RL_Bus.LM_RL_Line02.pC1
  Bus Selector4 : BusSelector  OutputSignals=TOS_LM_LR_Bus.LM_LR_Line02.dDisStart,TOS_LM_LR_Bus.LM_LR_Line02.dDisEnd
  Gain{1..4} (4 alike) : Gain  Gain=0.5  ParamDataTypeStr=single  OutDataTypeStr=single
  EgoLaneCenterLine02 : Outport
  wires:
  Bus Selector/1 -> Add/1  "<pC0>"
  Add/1 -> Gain4/1
  Bus Selector/2 -> Add/2  "<pC0>"
  Bus Selector1/2 -> Add1/2  "<pC3>"
  Bus Selector3/2 -> Add3/2  "<pC1>"
  Add1/1 -> Gain1/1
  Bus Selector1/1 -> Add1/1  "<pC3>"
  Bus Selector2/2 -> Add2/2  "<pC2>"
  Add3/1 -> Gain3/1
  Bus Selector2/1 -> Add2/1  "<pC2>"
  EgoLaneLine/1 -> Bus Selector1/1, Bus Selector2/1, Bus Selector3/1, Bus Selector4/1, Bus Selector/1
  Bus Selector3/1 -> Add3/1  "<pC1>"
  Add2/1 -> Gain2/1
  Bus Creator/1 -> EgoLaneCenterLine02/1
  Gain4/1 -> Bus Creator/4  "PC0"
  Gain1/1 -> Bus Creator/1  "PC3"
  Gain2/1 -> Bus Creator/2  "PC2"
  Gain3/1 -> Bus Creator/3  "PC1"
  Bus Selector4/2 -> Bus Creator/6  "<dDisEnd>"
  Bus Selector4/1 -> Bus Creator/5  "<dDisStart>"

== system PubIfDecisionTOS_MDL/TOS_20201112/TOS_2012080320/PP1128/AAT-AdditionalAttributes/PP_ObjectToCenterLine_dy/EgoLaneCenterLine/EgoLaneCenterLine03 ==
  EgoLaneLine : Inport
  Add{,1..3} (4 alike) : Sum
  Bus Creator1 : BusCreator  Inputs=6
  Bus Selector : BusSelector  OutputSignals=TOS_LM_LR_Bus.LM_LR_Line03.pC0,TOS_LM_RL_Bus.LM_RL_Line03.pC0
  Bus Selector1 : BusSelector  OutputSignals=TOS_LM_LR_Bus.LM_LR_Line03.pC3,TOS_LM_RL_Bus.LM_RL_Line03.pC3
  Bus Selector2 : BusSelector  OutputSignals=TOS_LM_LR_Bus.LM_LR_Line03.pC2,TOS_LM_RL_Bus.LM_RL_Line03.pC2
  Bus Selector3 : BusSelector  OutputSignals=TOS_LM_LR_Bus.LM_LR_Line03.pC1,TOS_LM_RL_Bus.LM_RL_Line03.pC1
  Bus Selector4 : BusSelector  OutputSignals=TOS_LM_LR_Bus.LM_LR_Line03.dDisStart,TOS_LM_LR_Bus.LM_LR_Line03.dDisEnd
  Gain{1..4} (4 alike) : Gain  Gain=0.5  ParamDataTypeStr=single  OutDataTypeStr=single
  EgoLaneCenterLine03 : Outport
  wires:
  Bus Selector/2 -> Add/2  "<pC0>"
  Add/1 -> Gain4/1
  Bus Selector/1 -> Add/1  "<pC0>"
  Bus Selector1/2 -> Add1/2  "<pC3>"
  Bus Selector3/2 -> Add3/2  "<pC1>"
  Add1/1 -> Gain1/1
  Bus Selector1/1 -> Add1/1  "<pC3>"
  Bus Selector2/2 -> Add2/2  "<pC2>"
  Add3/1 -> Gain3/1
  Bus Selector2/1 -> Add2/1  "<pC2>"
  EgoLaneLine/1 -> Bus Selector1/1, Bus Selector2/1, Bus Selector3/1, Bus Selector4/1, Bus Selector/1
  Bus Selector3/1 -> Add3/1  "<pC1>"
  Add2/1 -> Gain2/1
  Bus Creator1/1 -> EgoLaneCenterLine03/1
  Gain4/1 -> Bus Creator1/4  "PC0"
  Gain1/1 -> Bus Creator1/1  "PC3"
  Gain2/1 -> Bus Creator1/2  "PC2"
  Gain3/1 -> Bus Creator1/3  "PC1"
  Bus Selector4/2 -> Bus Creator1/6  "<dDisEnd>"
  Bus Selector4/1 -> Bus Creator1/5  "<dDisStart>"

== system PubIfDecisionTOS_MDL/TOS_20201112/TOS_2012080320/PP1128/AAT-AdditionalAttributes/PP_ObjectToCenterLine_dy/EgoLaneCenterLine/EgoLaneCenterLine04 ==
  EgoLaneLine : Inport
  Add{,1..3} (4 alike) : Sum
  Bus Creator1 : BusCreator  Inputs=6
  Bus Selector : BusSelector  OutputSignals=TOS_LM_LR_Bus.LM_LR_Line04.pC0,TOS_LM_RL_Bus.LM_RL_Line04.pC0
  Bus Selector1 : BusSelector  OutputSignals=TOS_LM_LR_Bus.LM_LR_Line04.pC3,TOS_LM_RL_Bus.LM_RL_Line04.pC3
  Bus Selector2 : BusSelector  OutputSignals=TOS_LM_LR_Bus.LM_LR_Line04.pC2,TOS_LM_RL_Bus.LM_RL_Line04.pC2
  Bus Selector3 : BusSelector  OutputSignals=TOS_LM_LR_Bus.LM_LR_Line04.pC1,TOS_LM_RL_Bus.LM_RL_Line04.pC1
  Bus Selector4 : BusSelector  OutputSignals=TOS_LM_LR_Bus.LM_LR_Line04.dDisStart,TOS_LM_LR_Bus.LM_LR_Line04.dDisEnd
  Gain{1..4} (4 alike) : Gain  Gain=0.5  ParamDataTypeStr=single  OutDataTypeStr=single
  EgoLaneCenterLine04 : Outport
  wires:
  Bus Selector/1 -> Add/1  "<pC0>"
  Add/1 -> Gain4/1
  Bus Selector/2 -> Add/2  "<pC0>"
  Bus Selector1/2 -> Add1/2  "<pC3>"
  Bus Selector3/2 -> Add3/2  "<pC1>"
  Add1/1 -> Gain1/1
  Bus Selector1/1 -> Add1/1  "<pC3>"
  Bus Selector2/2 -> Add2/2  "<pC2>"
  Add3/1 -> Gain3/1
  Bus Selector2/1 -> Add2/1  "<pC2>"
  EgoLaneLine/1 -> Bus Selector1/1, Bus Selector2/1, Bus Selector3/1, Bus Selector4/1, Bus Selector/1
  Bus Selector3/1 -> Add3/1  "<pC1>"
  Add2/1 -> Gain2/1
  Gain4/1 -> Bus Creator1/4  "PC0"
  Gain1/1 -> Bus Creator1/1  "PC3"
  Gain2/1 -> Bus Creator1/2  "PC2"
  Gain3/1 -> Bus Creator1/3  "PC1"
  Bus Creator1/1 -> EgoLaneCenterLine04/1
  Bus Selector4/2 -> Bus Creator1/6  "<dDisEnd>"
  Bus Selector4/1 -> Bus Creator1/5  "<dDisStart>"

== system PubIfDecisionTOS_MDL/TOS_20201112/TOS_2012080320/PP1128/AAT-AdditionalAttributes/PP_ObjectToCenterLine_dy/EgoLaneCenterLine/EgoLaneCenterLine05 ==
  EgoLaneLine : Inport
  Add{,1..3} (4 alike) : Sum
  Bus Creator1 : BusCreator  Inputs=6
  Bus Selector : BusSelector  OutputSignals=TOS_LM_LR_Bus.LM_LR_Line05.pC0,TOS_LM_RL_Bus.LM_RL_Line05.pC0
  Bus Selector1 : BusSelector  OutputSignals=TOS_LM_LR_Bus.LM_LR_Line05.pC3,TOS_LM_RL_Bus.LM_RL_Line05.pC3
  Bus Selector2 : BusSelector  OutputSignals=TOS_LM_LR_Bus.LM_LR_Line05.pC2,TOS_LM_RL_Bus.LM_RL_Line05.pC2
  Bus Selector3 : BusSelector  OutputSignals=TOS_LM_LR_Bus.LM_LR_Line05.pC1,TOS_LM_RL_Bus.LM_RL_Line05.pC1
  Bus Selector4 : BusSelector  OutputSignals=TOS_LM_LR_Bus.LM_LR_Line05.dDisStart,TOS_LM_LR_Bus.LM_LR_Line05.dDisEnd
  Gain{1..4} (4 alike) : Gain  Gain=0.5  ParamDataTypeStr=single  OutDataTypeStr=single
  EgoLaneCenterLine05 : Outport
  wires:
  Bus Selector/1 -> Add/1  "<pC0>"
  Add/1 -> Gain4/1
  Bus Selector/2 -> Add/2  "<pC0>"
  Bus Selector1/2 -> Add1/2  "<pC3>"
  Add1/1 -> Gain1/1
  Bus Selector1/1 -> Add1/1  "<pC3>"
  Bus Selector2/2 -> Add2/2  "<pC2>"
  Add3/1 -> Gain3/1
  Bus Selector2/1 -> Add2/1  "<pC2>"
  Bus Selector3/1 -> Add3/1  "<pC1>"
  Add2/1 -> Gain2/1
  Bus Selector3/2 -> Add3/2  "<pC1>"
  Gain4/1 -> Bus Creator1/4  "PC0"
  Gain1/1 -> Bus Creator1/1  "PC3"
  Gain2/1 -> Bus Creator1/2  "PC2"
  Gain3/1 -> Bus Creator1/3  "PC1"
  Bus Creator1/1 -> EgoLaneCenterLine05/1
  Bus Selector4/1 -> Bus Creator1/5  "<dDisStart>"
  EgoLaneLine/1 -> Bus Selector1/1, Bus Selector2/1, Bus Selector3/1, Bus Selector4/1, Bus Selector/1
  Bus Selector4/2 -> Bus Creator1/6  "<dDisEnd>"

== system PubIfDecisionTOS_MDL/TOS_20201112/TOS_2012080320/PP1128/AAT-AdditionalAttributes/PP_ObjectToCenterLine_dy/EgoLaneCenterLine/EgoLaneCenterLine06 ==
  EgoLaneLine : Inport
  Add{,1..3} (4 alike) : Sum
  Bus Creator1 : BusCreator  Inputs=6
  Bus Selector : BusSelector  OutputSignals=TOS_LM_LR_Bus.LM_LR_Line06.pC0,TOS_LM_RL_Bus.LM_RL_Line06.pC0
  Bus Selector1 : BusSelector  OutputSignals=TOS_LM_LR_Bus.LM_LR_Line06.pC3,TOS_LM_RL_Bus.LM_RL_Line06.pC3
  Bus Selector2 : BusSelector  OutputSignals=TOS_LM_LR_Bus.LM_LR_Line06.pC2,TOS_LM_RL_Bus.LM_RL_Line06.pC2
  Bus Selector3 : BusSelector  OutputSignals=TOS_LM_LR_Bus.LM_LR_Line06.pC1,TOS_LM_RL_Bus.LM_RL_Line06.pC1
  Bus Selector4 : BusSelector  OutputSignals=TOS_LM_LR_Bus.LM_LR_Line06.dDisStart,TOS_LM_LR_Bus.LM_LR_Line06.dDisEnd
  Gain{1..4} (4 alike) : Gain  Gain=0.5  ParamDataTypeStr=single  OutDataTypeStr=single
  EgoLaneCenterLine06 : Outport
  wires:
  Bus Selector/1 -> Add/1  "<pC0>"
  Add/1 -> Gain4/1
  Bus Selector/2 -> Add/2  "<pC0>"
  Bus Selector1/2 -> Add1/2  "<pC3>"
  Bus Selector3/2 -> Add3/2  "<pC1>"
  Add1/1 -> Gain1/1
  Bus Selector1/1 -> Add1/1  "<pC3>"
  Bus Selector2/2 -> Add2/2  "<pC2>"
  Add3/1 -> Gain3/1
  Bus Selector2/1 -> Add2/1  "<pC2>"
  Bus Selector3/1 -> Add3/1  "<pC1>"
  Add2/1 -> Gain2/1
  Gain4/1 -> Bus Creator1/4  "PC0"
  Gain1/1 -> Bus Creator1/1  "PC3"
  Gain2/1 -> Bus Creator1/2  "PC2"
  Gain3/1 -> Bus Creator1/3  "PC1"
  Bus Creator1/1 -> EgoLaneCenterLine06/1
  EgoLaneLine/1 -> Bus Selector1/1, Bus Selector2/1, Bus Selector3/1, Bus Selector4/1, Bus Selector/1
  Bus Selector4/1 -> Bus Creator1/5  "<dDisStart>"
  Bus Selector4/2 -> Bus Creator1/6  "<dDisEnd>"

== system PubIfDecisionTOS_MDL/TOS_20201112/TOS_2012080320/PP1128/AAT-AdditionalAttributes/PP_ObjectToCenterLine_dy/PP_EgoVeh_Object_ToCenterLine/EgoVehCenterLine_dy ==
  EgoVehCenterLine_dy : Inport
  Gain : Gain  Gain=-1  OutDataTypeStr=single
  PP_EgoVehCenterLine_dy : Outport
  wires:
  EgoVehCenterLine_dy/1 -> Gain/1
  Gain/1 -> PP_EgoVehCenterLine_dy/1

== system PubIfDecisionTOS_MDL/TOS_20201112/TOS_2012080320/PP1128/AAT-AdditionalAttributes/PP_ObjectToCenterLine_dy/PP_EgoVeh_Object_ToCenterLine/PP_ObjectToCenterLine ==
  TOS_OFMObjValid_Flag : Inport  Partition=on  PartitionDimension=1  PartitionWidth=1  PartitionOffset=0
  Object_DY : Inport  Port=2  Partition=on  PartitionDimension=1  PartitionWidth=1  PartitionOffset=0
  Object_DX : Inport  Port=3  Partition=on  PartitionDimension=1  PartitionWidth=1  PartitionOffset=0
  line01_C0 : Inport  Port=4
  line01_C1 : Inport  Port=5
  line01_C2 : Inport  Port=6
  line01_C3 : Inport  Port=7
  line01_dDisStart : Inport  Port=8
  line01_dDisEnd : Inport  Port=9
  line02_C0 : Inport  Port=10
  line02_C1 : Inport  Port=11
  line02_C2 : Inport  Port=12
  line02_C3 : Inport  Port=13
  line02_dDisStart : Inport  Port=14
  line02_dDisEnd : Inport  Port=15
  line03_C0 : Inport  Port=16
  line03_C1 : Inport  Port=17
  line03_C2 : Inport  Port=18
  line03_C3 : Inport  Port=19
  line03_dDisStart : Inport  Port=20
  line03_dDisEnd : Inport  Port=21
  line04_C0 : Inport  Port=22
  line04_C1 : Inport  Port=23
  line04_C2 : Inport  Port=24
  line04_C3 : Inport  Port=25
  line04_dDisStart : Inport  Port=26
  line04_dDisEnd : Inport  Port=27
  line05_C0 : Inport  Port=28
  line05_C1 : Inport  Port=29
  line05_C2 : Inport  Port=30
  line05_C3 : Inport  Port=31
  line05_dDisStart : Inport  Port=32
  line05_dDisEnd : Inport  Port=33
  line06_C0 : Inport  Port=34
  line06_C1 : Inport  Port=35
  line06_C2 : Inport  Port=36
  line06_C3 : Inport  Port=37
  line06_dDisStart : Inport  Port=38
  line06_dDisEnd : Inport  Port=39
  Compare To Constant : simulink/Logic and Bit Operations/Compare To Constant  relop===  const=C_TOS_OFMObjIDInvilad_Val  OutDataTypeStr=boolean
      settings: AttributesFormatString=C_TOS_OFMObjIDInvilad_Val = 0
  For Each : ForEach  DisableCoverage=on
  If : If  IfExpression=u1 ~= 0
  Merge : Merge
  PP_ObjectToCenterLineDefault : Subsystem  TreatAsAtomicUnit=on
  PP_ObjectToCenterLine_ : Subsystem
  PP_ObjectToCenterLine_dy : Outport  ConcatenationDimension=1
  wires:
  Object_DY/1 -> PP_ObjectToCenterLine_/1(Object_DY)
  Object_DX/1 -> PP_ObjectToCenterLine_/2(Object_DX)
  line01_C0/1 -> PP_ObjectToCenterLine_/3(line01_C0)
  line01_C1/1 -> PP_ObjectToCenterLine_/4(line01_C1)
  line01_C2/1 -> PP_ObjectToCenterLine_/5(line01_C2)
  line01_C3/1 -> PP_ObjectToCenterLine_/6(line01_C3)
  line01_dDisStart/1 -> PP_ObjectToCenterLine_/7(line01_dDisStart)
  line01_dDisEnd/1 -> PP_ObjectToCenterLine_/8(line01_dDisEnd)
  line02_C0/1 -> PP_ObjectToCenterLine_/9(line02_C0)
  line02_C1/1 -> PP_ObjectToCenterLine_/10(line02_C1)
  line02_C2/1 -> PP_ObjectToCenterLine_/11(line02_C2)
  line02_C3/1 -> PP_ObjectToCenterLine_/12(line02_C3)
  line02_dDisStart/1 -> PP_ObjectToCenterLine_/13(line02_dDisStart)
  line02_dDisEnd/1 -> PP_ObjectToCenterLine_/14(line02_dDisEnd)
  line03_C0/1 -> PP_ObjectToCenterLine_/15(line03_C0)
  line03_C1/1 -> PP_ObjectToCenterLine_/16(line03_C1)
  line03_C2/1 -> PP_ObjectToCenterLine_/17(line03_C2)
  line03_C3/1 -> PP_ObjectToCenterLine_/18(line03_C3)
  line03_dDisStart/1 -> PP_ObjectToCenterLine_/19(line03_dDisStart)
  line03_dDisEnd/1 -> PP_ObjectToCenterLine_/20(line03_dDisEnd)
  line04_C0/1 -> PP_ObjectToCenterLine_/21(line04_C0)
  line04_C1/1 -> PP_ObjectToCenterLine_/22(line04_C1)
  line04_C2/1 -> PP_ObjectToCenterLine_/23(line04_C2)
  line04_C3/1 -> PP_ObjectToCenterLine_/24(line04_C3)
  line04_dDisStart/1 -> PP_ObjectToCenterLine_/25(line04_dDisStart)
  line04_dDisEnd/1 -> PP_ObjectToCenterLine_/26(line04_dDisEnd)
  line05_C0/1 -> PP_ObjectToCenterLine_/27(line05_C0)
  line05_C1/1 -> PP_ObjectToCenterLine_/28(line05_C1)
  line05_C2/1 -> PP_ObjectToCenterLine_/29(line05_C2)
  line05_C3/1 -> PP_ObjectToCenterLine_/30(line05_C3)
  line05_dDisStart/1 -> PP_ObjectToCenterLine_/31(line05_dDisStart)
  line05_dDisEnd/1 -> PP_ObjectToCenterLine_/32(line05_dDisEnd)
  line06_C0/1 -> PP_ObjectToCenterLine_/33(line06_C0)
  line06_C1/1 -> PP_ObjectToCenterLine_/34(line06_C1)
  line06_C2/1 -> PP_ObjectToCenterLine_/35(line06_C2)
  line06_C3/1 -> PP_ObjectToCenterLine_/36(line06_C3)
  line06_dDisStart/1 -> PP_ObjectToCenterLine_/37(line06_dDisStart)
  line06_dDisEnd/1 -> PP_ObjectToCenterLine_/38(line06_dDisEnd)
  PP_ObjectToCenterLine_/1(PP_ObjectToCenterLine_dy) -> Merge/2
  If/1 -> PP_ObjectToCenterLineDefault/Action
  Compare To Constant/1 -> If/1
  If/2 -> PP_ObjectToCenterLine_/Action
  TOS_OFMObjValid_Flag/1 -> Compare To Constant/1
  Merge/1 -> PP_ObjectToCenterLine_dy/1
  PP_ObjectToCenterLineDefault/1(PP_ObjectToCenterLine_dy) -> Merge/1
